simulink model "Control_Seminar"  (R2022b)
settings: Solver=VariableStepAuto  StartTime=0.0  StopTime=10.0  MaxStep=0.01  RelTol=1e-3
settings Model: Creator=15043  LastModifiedBy=15043

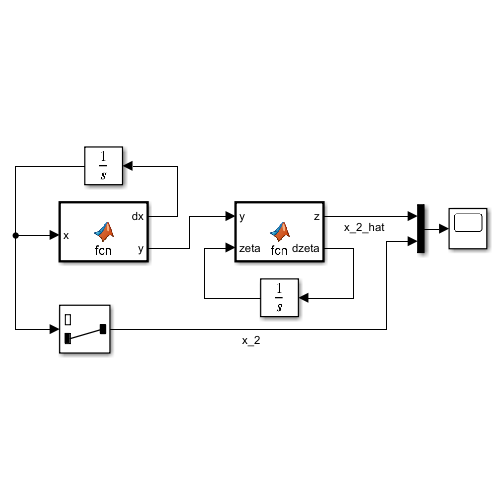
[thumbnail: Simulink's stored preview of the top-level diagram]
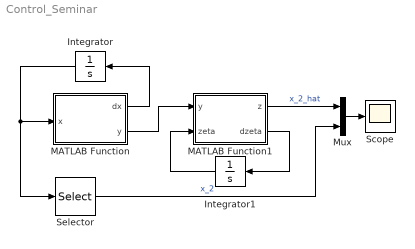
== system Control_Seminar ==
  Integrator : Integrator  InitialCondition=[0.01;0]
  Integrator1 : Integrator  InitialCondition=0.1
  MATLAB Function : MATLAB Function  TreatAsAtomicUnit=on
  MATLAB Function1 : MATLAB Function  TreatAsAtomicUnit=on
  Mux : Mux  Inputs=2
  Scope : Scope
  Selector : Selector  InputPortWidth=2  IndexOptions=Index vector (dialog)  Indices=[2]  OutputSizes=1
  wires:
  MATLAB Function/1(dx) -> Integrator/1
  Integrator/1 -> Selector/1, MATLAB Function/1(x)
  MATLAB Function/2(y) -> MATLAB Function1/1(y)
  MATLAB Function1/2(dzeta) -> Integrator1/1
  Integrator1/1 -> MATLAB Function1/2(zeta)
  Mux/1 -> Scope/1
  MATLAB Function1/1(z) -> Mux/1  "x_2_hat"
  Selector/1 -> Mux/2  "x_2"

== matlab function Control_Seminar/MATLAB Function ==
  data: dx output; x input; y output
function [dx, y] = pendulum(x)
w0 = 3;

x1 = x(1);
x2 = x(2);

dx1 = x2;
dx2 = -sin(x1*w0^2);

dx = [dx1; dx2];
y = x1;

== matlab function Control_Seminar/MATLAB Function1 ==
  data: z output; y input; dzeta output; zeta input
function [z, dzeta] = obs(y, zeta)
w0 = 3;
dzeta = -sin(y*w0^2) - 5*w0*(zeta + 5*w0*y);
z = zeta + 5*w0*y;
